simulink library "hil14_mdl_lib"  (Simulink 7.0)
values from neighbouring files (symbols this model uses):
  air =     [ws.mat]
  amb =     [ws.mat]
  cylinder =     [ws.mat]
  fuel =     [ws.mat]
  im =     [ws.mat]
  MDL =     [ws.mat]
  mph_per_m_per_sec = 2.23713646532    [ws.mat]
  tc =     [ws.mat]
  trans =     [ws.mat]
  veh =     [ws.mat]
  whl =     [ws.mat]
libraries: ni_annotations_lib x13
settings Model: Creator=Eric Bradley  LastModifiedBy=Eric Bradley

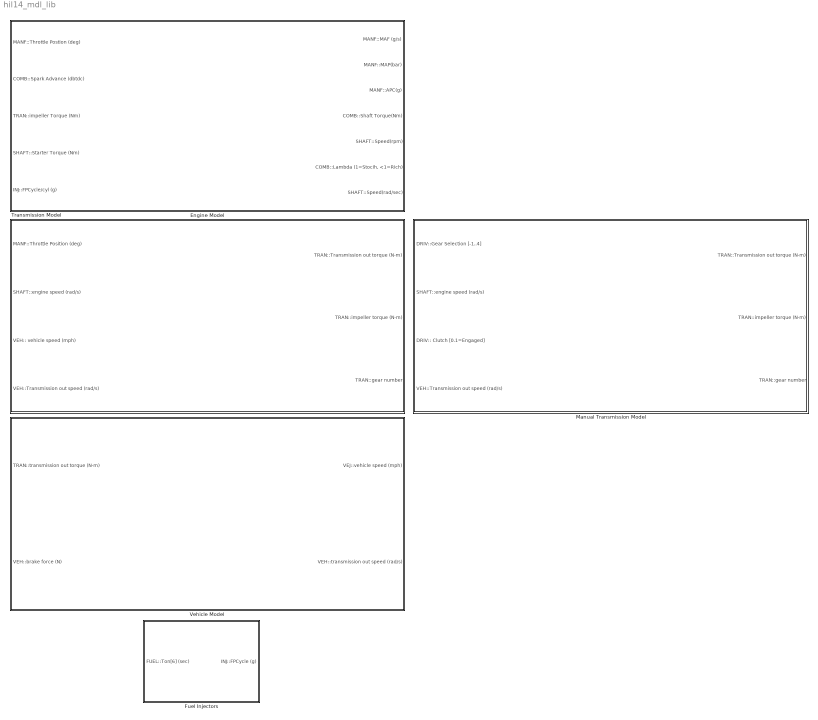
== system hil14_mdl_lib ==
  Engine Model : Subsystem  mask{iname='engine.jpg'}
      mask prompts: iname "Image"
      mask init:
      | blk = gcb;
      | 
      | p = get_param(blk,'Position');
      | 
      | wd = p(3)-p(1);
      | ht = p(4)-p(2);
      | 
      | ar = wd/ht;
      | 
      | img = imread(iname);
      | ii = imfinfo(iname);
      | 
      | iar = ii.Width/ii.Height;
      | 
      | scale = 0.125;
      settings: OpenFcn=open_system(gcb,'Force')
      mask Display: image(img, [0.5-ii.Width/wd*scale/2, 0.5-ii.Height/ht*scale/2, ii.Width/wd*scale,ii.Height/ht*scale]);
  Fuel Injectors : Subsystem  mask{iname='pfi.jpg', scale=0.125}
      mask prompts: iname "Image"
      mask init:
      | blk = gcb;
      | 
      | p = get_param(blk,'Position');
      | 
      | wd = p(3)-p(1);
      | ht = p(4)-p(2);
      | 
      | ar = wd/ht;
      | 
      | img = imread(iname);
      | ii = imfinfo(iname);
      | 
      | iar = ii.Width/ii.Height;
      settings: OpenFcn=open_system(gcb,'Force')
      mask Display: image(img, [0.5-ii.Width/wd*scale/2, 0.5-ii.Height/ht*scale/2, ii.Width/wd*scale,ii.Height/ht*scale]);
  Manual Transmission Model : Subsystem  mask{iname='Manual_Transmission.png', scale=0.55}
      mask prompts: iname "Image"
      mask init:
      | blk = gcb;
      | 
      | p = get_param(blk,'Position');
      | 
      | wd = p(3)-p(1);
      | ht = p(4)-p(2);
      | 
      | ar = wd/ht;
      | 
      | img = imread(iname);
      | ii = imfinfo(iname);
      | 
      | iar = ii.Width/ii.Height;
      settings: OpenFcn=open_system(gcb,'Force')
      mask Display: image(img, [0.5-ii.Width/wd*scale/2, 0.5-ii.Height/ht*scale/2, ii.Width/wd*scale,ii.Height/ht*scale]);
  Transmission Model : Subsystem  mask{iname='tran.jpg', scale=0.375}
      mask prompts: iname "Image"
      mask init:
      | blk = gcb;
      | 
      | p = get_param(blk,'Position');
      | 
      | wd = p(3)-p(1);
      | ht = p(4)-p(2);
      | 
      | ar = wd/ht;
      | 
      | img = imread(iname);
      | ii = imfinfo(iname);
      | 
      | iar = ii.Width/ii.Height;
      settings: OpenFcn=open_system(gcb,'Force')
      mask Display: image(img, [0.5-ii.Width/wd*scale/2, 0.5-ii.Height/ht*scale/2, ii.Width/wd*scale,ii.Height/ht*scale]);
  Vehicle Model : Subsystem  mask{iname='veh.jpg', scale=0.5}
      mask prompts: iname "Image"
      mask init:
      | blk = gcb;
      | 
      | p = get_param(blk,'Position');
      | 
      | wd = p(3)-p(1);
      | ht = p(4)-p(2);
      | 
      | ar = wd/ht;
      | 
      | img = imread(iname);
      | ii = imfinfo(iname);
      | 
      | iar = ii.Width/ii.Height;
      settings: OpenFcn=open_system(gcb,'Force')
      mask Display: image(img, [0.5-ii.Width/wd*scale/2, 0.5-ii.Height/ht*scale/2, ii.Width/wd*scale,ii.Height/ht*scale]);

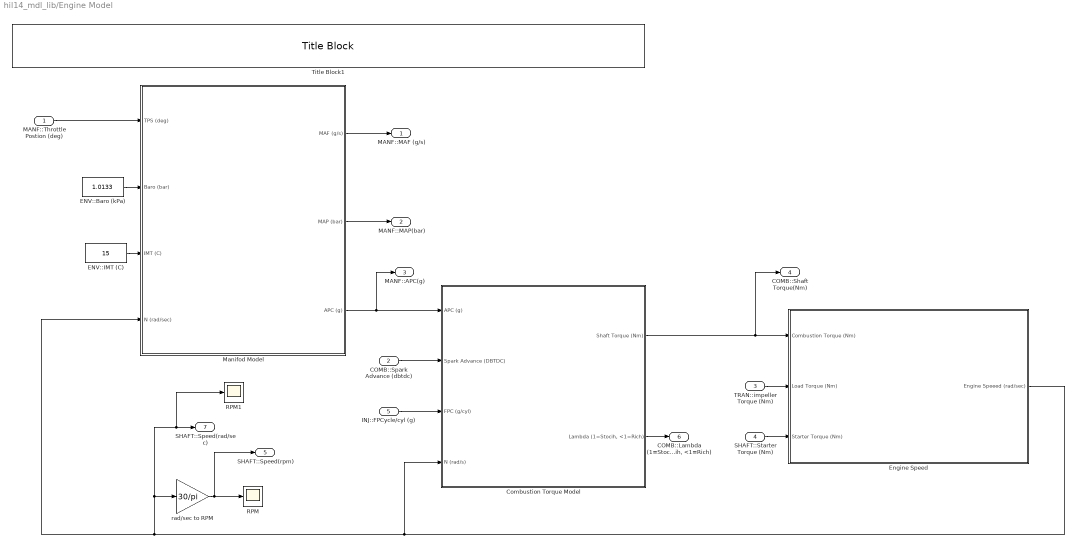
== system hil14_mdl_lib/Engine Model ==
  MANF::Throttle Postion (deg) : Inport  OutDataType=sfix(16)  OutScaling=2^0
  COMB::Spark Advance (dbtdc) : Inport  Port=2  PortDimensions=6  OutDataType=sfix(16)  OutScaling=2^0
  TRAN::impeller Torque (Nm) : Inport  Port=3  OutDataType=sfix(16)  OutScaling=2^0
  SHAFT::Starter Torque (Nm) : Inport  Port=4  OutDataType=sfix(16)  OutScaling=2^0
  INJ::FPCycle/cyl (g) : Inport  Port=5  OutDataType=sfix(16)  OutScaling=2^0
  Combustion Torque Model : Subsystem  mask{iname='cylinder.jpg'}
      mask prompts: iname "Image"
      mask init:
      | blk = gcb;
      | 
      | p = get_param(blk,'Position');
      | 
      | wd = p(3)-p(1);
      | ht = p(4)-p(2);
      | 
      | ar = wd/ht;
      | 
      | img = imread(iname);
      | ii = imfinfo(iname);
      | 
      | iar = ii.Width/ii.Height;
      settings: OpenFcn=open_system(gcb,'Force')
      mask Display: image(img, [0.5-ii.Width/wd*0.125/2, 0.5-ii.Height/ht*0.125/2, ii.Width/wd*0.125,ii.Height/ht*0.125]);
  ENV::Baro (kPa) : Constant  Value=1.0133  OutDataType=sfix(16)  OutScaling=2^0
  ENV::IMT (C) : Constant  Value=15  OutDataType=sfix(16)  OutScaling=2^0
  Engine Speed : Subsystem  mask{iname='piston.jpg'}
      mask prompts: iname "Image"
      mask init:
      | blk = gcb;
      | 
      | p = get_param(blk,'Position');
      | 
      | wd = p(3)-p(1);
      | ht = p(4)-p(2);
      | 
      | ar = wd/ht;
      | 
      | img = imread(iname);
      | ii = imfinfo(iname);
      | 
      | iar = ii.Width/ii.Height;
      settings: OpenFcn=open_system(gcb,'Force')
      mask Display: image(img, [0.5-ii.Width/wd*0.5/2, 0.5-ii.Height/ht*0.5/2, ii.Width/wd*0.5,ii.Height/ht*0.5]);
  Manifod Model : Subsystem  mask{iname='intake_manifold.jpg'}
      mask prompts: iname "Image"
      mask init:
      | blk = gcb;
      | 
      | p = get_param(blk,'Position');
      | 
      | wd = p(3)-p(1);
      | ht = p(4)-p(2);
      | 
      | ar = wd/ht;
      | 
      | img = imread(iname);
      | ii = imfinfo(iname);
      | 
      | iar = ii.Width/ii.Height;
      settings: OpenFcn=open_system(gcb,'Force')
      mask Display: image(img, [0.5-ii.Width/wd*0.25/2, 0.5-ii.Height/ht*0.25/2, ii.Width/wd*0.25,ii.Height/ht*0.25]);
  RPM : Scope
      settings: YMin=1100  YMax=2200  SaveName=ScopeData8
  RPM1 : Scope
      settings: YMin=1100  YMax=2200  SaveName=ScopeData14
  Title Block1 : ni_annotations_lib/Title Block  SystemSampleTime=-1  tx_title=get_param(gcs,'Name')
  rad/sec to RPM : Gain  Gain=30/pi  ParameterDataType=sfix(16)  ParameterScaling=2^0  OutDataType=sfix(16)  OutScaling=2^0
  MANF::MAF (g/s) : Outport  OutDataType=sfix(16)  OutScaling=2^0
  MANF::MAP(bar) : Outport  Port=2  OutDataType=sfix(16)  OutScaling=2^0
  MANF::APC(g) : Outport  Port=3  OutDataType=sfix(16)  OutScaling=2^0
  COMB::Shaft Torque(Nm) : Outport  Port=4  OutDataType=sfix(16)  OutScaling=2^0
  SHAFT::Speed(rpm) : Outport  Port=5  OutDataType=sfix(16)  OutScaling=2^0
  "COMB::Lambda (1=Stocih, <1=Rich)" : Outport  Port=6  OutDataType=sfix(16)  OutScaling=2^0
  SHAFT::Speed(rad/sec) : Outport  Port=7  OutDataType=sfix(16)  OutScaling=2^0
  wires:
  INJ::FPCycle/cyl (g)/1 -> Combustion Torque Model/3(FPC (g/cyl))
  SHAFT::Starter Torque (Nm)/1 -> Engine Speed/3(Starter Torque (Nm))
  TRAN::impeller Torque (Nm)/1 -> Engine Speed/2(Load Torque (Nm))
  COMB::Spark Advance (dbtdc)/1 -> Combustion Torque Model/2(Spark Advance (DBTDC))
  Combustion Torque Model/2("Lambda (1=Stocih, <1=Rich)") -> "COMB::Lambda (1=Stocih, <1=Rich)"/1
  MANF::Throttle Postion (deg)/1 -> Manifod Model/1(TPS (deg))
  Engine Speed/1(Engine Speeed (rad/sec)) -> Combustion Torque Model/4(N (rad/s)), RPM1/1, SHAFT::Speed(rad/sec)/1, rad/sec to RPM/1, Manifod Model/4(N (rad/sec))
  rad/sec to RPM/1 -> SHAFT::Speed(rpm)/1, RPM/1
  Combustion Torque Model/1(Shaft Torque (Nm)) -> COMB::Shaft Torque(Nm)/1, Engine Speed/1(Combustion Torque (Nm))
  Manifod Model/3(APC (g)) -> Combustion Torque Model/1(APC (g)), MANF::APC(g)/1
  Manifod Model/2(MAP (bar)) -> MANF::MAP(bar)/1
  Manifod Model/1(MAF (g/s)) -> MANF::MAF (g/s)/1
  ENV::IMT (C)/1 -> Manifod Model/3(IMT (C))
  ENV::Baro (kPa)/1 -> Manifod Model/2(Baro (bar))

== system hil14_mdl_lib/Fuel Injectors ==
  FUEL::Ton[6] (sec) : Inport  PortDimensions=6  OutDataType=sfix(16)  OutScaling=2^0
  Injector Curve : Lookup  InputValues=MDL.ECU_ENGINE.InjectionTime.v(14,:)'  Table=MDL.ECU_ENGINE.InjectionTime.y*1000  LookUpMeth=Interpolation-Use End Values  OutDataTypeMode=double  OutDataType=sfix(16)  OutScaling=2^0
  Sum of Elements : Sum  Inputs=+  OutDataType=sfix(16)  OutScaling=2^-10
  Title Block1 : ni_annotations_lib/Title Block  SystemSampleTime=-1  tx_title=get_param(gcs,'Name')
  INJ::FPCycle (g) : Outport  OutDataType=sfix(16)  OutScaling=2^0
  wires:
  Sum of Elements/1 -> INJ::FPCycle (g)/1
  Injector Curve/1 -> Sum of Elements/1
  FUEL::Ton[6] (sec)/1 -> Injector Curve/1

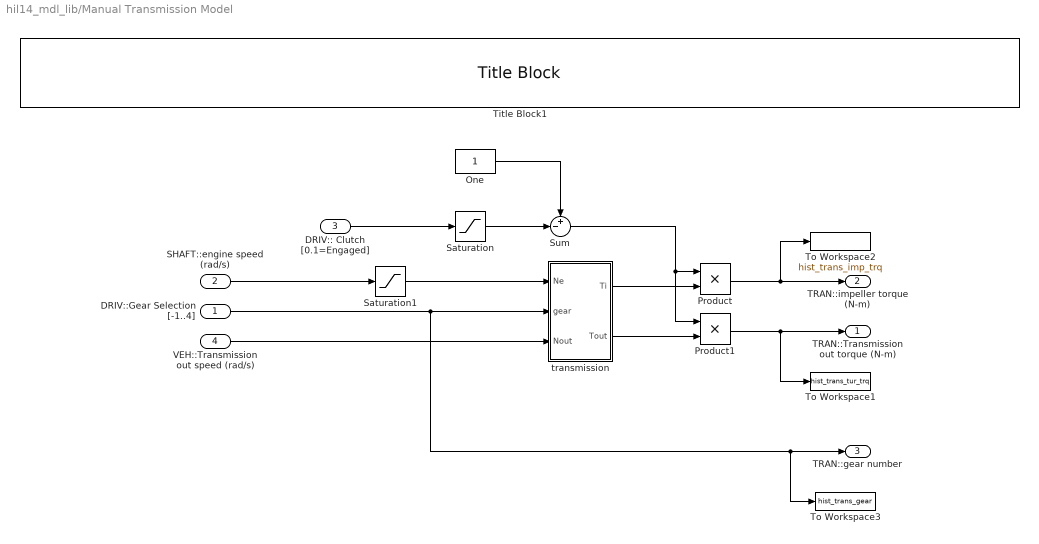
== system hil14_mdl_lib/Manual Transmission Model ==
  DRIV::Gear Selection [-1..4] : Inport  OutDataType=sfix(16)  OutScaling=2^0
  SHAFT::engine speed (rad/s) : Inport  Port=2  OutDataType=sfix(16)  OutScaling=2^0
  DRIV:: Clutch [0.1=Engaged] : Inport  Port=3  OutDataType=sfix(16)  OutScaling=2^0
  VEH::Transmission out speed (rad/s) : Inport  Port=4  OutDataType=sfix(16)  OutScaling=2^0
  One : Constant  OutDataType=sfix(16)  OutScaling=2^0
  Product : Product  OutDataType=sfix(16)  OutScaling=2^0  RndMeth=Zero
  Product1 : Product  OutDataType=sfix(16)  OutScaling=2^0  RndMeth=Zero
  Saturation : Saturate  UpperLimit=1  LowerLimit=0  OutDataType=sfix(16)  OutScaling=2^0
  Saturation1 : Saturate  UpperLimit=inf  LowerLimit=2*pi/60  OutDataType=sfix(16)  OutScaling=2^0
  Sum : Sum  Inputs=+-|  OutDataType=sfix(16)  OutScaling=2^0
  Title Block1 : ni_annotations_lib/Title Block  SystemSampleTime=-1  tx_title=get_param(gcs,'Name')
  To Workspace1 : ToWorkspace  VariableName=hist_trans_tur_trq  SampleTime=-1  SaveFormat=Array
      settings: MaxDataPoints=hist_sample_size
  To Workspace2 : ToWorkspace  VariableName=hist_trans_imp_trq  SampleTime=-1  SaveFormat=Array
      settings: MaxDataPoints=hist_sample_size
  To Workspace3 : ToWorkspace  VariableName=hist_trans_gear  SampleTime=-1  SaveFormat=Array
      settings: MaxDataPoints=hist_sample_size
  transmission : Subsystem
  TRAN::Transmission out torque (N-m) : Outport  InitialOutput=0
  TRAN::impeller torque (N-m) : Outport  Port=2  InitialOutput=0
  TRAN::gear number : Outport  Port=3  InitialOutput=0
  wires:
  Saturation1/1 -> transmission/1(Ne)
  Sum/1 -> Product1/1, Product/1
  One/1 -> Sum/1
  Saturation/1 -> Sum/2
  Product1/1 -> To Workspace1/1, TRAN::Transmission out torque (N-m)/1
  transmission/2(Tout) -> Product1/2
  transmission/1(Ti) -> Product/2
  Product/1 -> To Workspace2/1, TRAN::impeller torque (N-m)/1
  DRIV:: Clutch [0.1=Engaged]/1 -> Saturation/1
  DRIV::Gear Selection [-1..4]/1 -> To Workspace3/1, TRAN::gear number/1, transmission/2(gear)
  VEH::Transmission out speed (rad/s)/1 -> transmission/3(Nout)
  SHAFT::engine speed (rad/s)/1 -> Saturation1/1

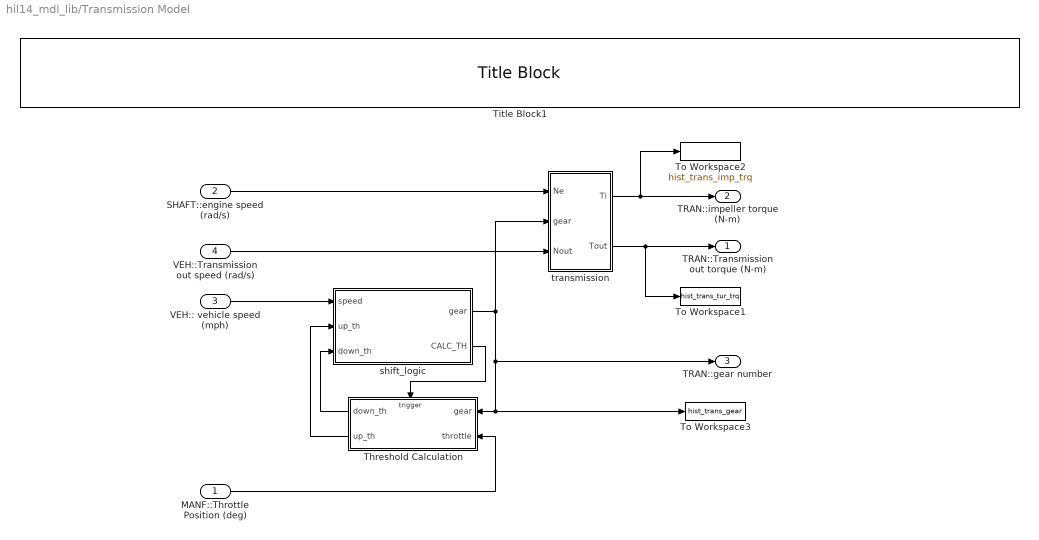
== system hil14_mdl_lib/Transmission Model ==
  MANF::Throttle Position (deg) : Inport  OutDataType=sfix(16)  OutScaling=2^0
  SHAFT::engine speed (rad/s) : Inport  Port=2  OutDataType=sfix(16)  OutScaling=2^0
  VEH:: vehicle speed (mph) : Inport  Port=3  OutDataType=sfix(16)  OutScaling=2^0
  VEH::Transmission out speed (rad/s) : Inport  Port=4  OutDataType=sfix(16)  OutScaling=2^0
  Threshold Calculation : Subsystem  Orientation=left  TreatAsAtomicUnit=on
  Title Block1 : ni_annotations_lib/Title Block  SystemSampleTime=-1  tx_title=get_param(gcs,'Name')
  To Workspace1 : ToWorkspace  VariableName=hist_trans_tur_trq  SampleTime=-1  SaveFormat=Array
      settings: MaxDataPoints=hist_sample_size
  To Workspace2 : ToWorkspace  VariableName=hist_trans_imp_trq  SampleTime=-1  SaveFormat=Array
      settings: MaxDataPoints=hist_sample_size
  To Workspace3 : ToWorkspace  VariableName=hist_trans_gear  SampleTime=-1  SaveFormat=Array
      settings: MaxDataPoints=hist_sample_size
  shift_logic : Stateflow chart
  transmission : Subsystem
  TRAN::Transmission out torque (N-m) : Outport  InitialOutput=0
  TRAN::impeller torque (N-m) : Outport  Port=2  InitialOutput=0
  TRAN::gear number : Outport  Port=3  InitialOutput=0
  wires:
  VEH::Transmission out speed (rad/s)/1 -> transmission/3(Nout)
  VEH:: vehicle speed (mph)/1 -> shift_logic/1(speed)
  transmission/1(Ti) -> TRAN::impeller torque (N-m)/1, To Workspace2/1
  MANF::Throttle Position (deg)/1 -> Threshold Calculation/2(throttle)
  SHAFT::engine speed (rad/s)/1 -> transmission/1(Ne)
  transmission/2(Tout) -> TRAN::Transmission out torque (N-m)/1, To Workspace1/1
  Threshold Calculation/1(down_th) -> shift_logic/3(down_th)
  Threshold Calculation/2(up_th) -> shift_logic/2(up_th)
  shift_logic/1(gear) -> transmission/2(gear), Threshold Calculation/1(gear), To Workspace3/1, TRAN::gear number/1
  shift_logic/2(CALC_TH) -> Threshold Calculation/Trigger

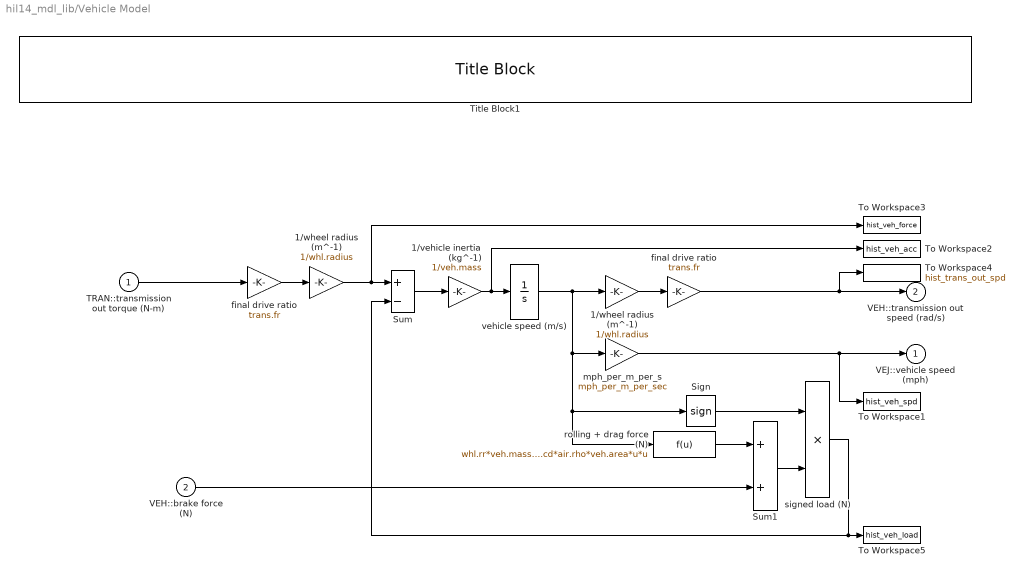
== system hil14_mdl_lib/Vehicle Model ==
  TRAN::transmission out torque (N-m) : Inport  OutDataType=sfix(16)  OutScaling=2^0
  VEH::brake force (N) : Inport  Port=2  OutDataType=sfix(16)  OutScaling=2^0
  1/vehicle inertia (kg^-1) : Gain  Gain=1/veh.mass  ParameterDataType=sfix(16)  ParameterScaling=2^0  OutDataType=sfix(16)  OutScaling=2^0  SaturateOnIntegerOverflow=on
  1/wheel radius (m^-1) : Gain  Gain=1/whl.radius  ParameterDataType=sfix(16)  ParameterScaling=2^0  OutDataType=sfix(16)  OutScaling=2^0  SaturateOnIntegerOverflow=on
  "1/wheel radius (m^-1) " : Gain  Gain=1/whl.radius  ParameterDataType=sfix(16)  ParameterScaling=2^0  OutDataType=sfix(16)  OutScaling=2^0  SaturateOnIntegerOverflow=on
  Sign : Signum
  Sum : Sum  Inputs=+-  OutDataType=sfix(16)  OutScaling=2^0  SaturateOnIntegerOverflow=on  InputSameDT=on
  Sum1 : Sum  OutDataType=sfix(16)  OutScaling=2^0  SaturateOnIntegerOverflow=on  InputSameDT=on
  Title Block1 : ni_annotations_lib/Title Block  SystemSampleTime=-1  tx_title=get_param(gcs,'Name')
  To Workspace1 : ToWorkspace  VariableName=hist_veh_spd  SampleTime=-1  SaveFormat=Array
      settings: MaxDataPoints=hist_sample_size
  To Workspace2 : ToWorkspace  VariableName=hist_veh_acc  SampleTime=-1  SaveFormat=Array
      settings: MaxDataPoints=hist_sample_size
  To Workspace3 : ToWorkspace  VariableName=hist_veh_force  SampleTime=-1  SaveFormat=Array
      settings: MaxDataPoints=hist_sample_size
  To Workspace4 : ToWorkspace  VariableName=hist_trans_out_spd  SampleTime=-1  SaveFormat=Array
      settings: MaxDataPoints=hist_sample_size
  To Workspace5 : ToWorkspace  VariableName=hist_veh_load  SampleTime=-1  SaveFormat=Array
      settings: MaxDataPoints=hist_sample_size
  final drive ratio : Gain  Gain=trans.fr  ParameterDataType=sfix(16)  ParameterScaling=2^0  OutDataType=sfix(16)  OutScaling=2^0  SaturateOnIntegerOverflow=on
  "final drive ratio " : Gain  Gain=trans.fr  ParameterDataType=sfix(16)  ParameterScaling=2^0  OutDataType=sfix(16)  OutScaling=2^0  SaturateOnIntegerOverflow=on
  mph_per_m_per_s : Gain  Gain=mph_per_m_per_sec  ParameterDataType=sfix(16)  ParameterScaling=2^0  OutDataType=sfix(16)  OutScaling=2^0  SaturateOnIntegerOverflow=on
  rolling + drag force (N) : Fcn  Expr=whl.rr*veh.mass*9.81 + 1/2*veh.cd*air.rho*veh.area*u*u
  signed load (N) : Product  OutDataType=sfix(16)  OutScaling=2^0  SaturateOnIntegerOverflow=on  InputSameDT=on
  vehicle speed (m/s) : Integrator  LowerSaturationLimit=0  ZeroCross=off
  VEJ::vehicle speed (mph) : Outport  InitialOutput=0
  VEH::transmission out speed (rad/s) : Outport  Port=2  InitialOutput=0
  wires:
  mph_per_m_per_s/1 -> To Workspace1/1, VEJ::vehicle speed (mph)/1
  "1/wheel radius (m^-1) "/1 -> "final drive ratio "/1
  signed load (N)/1 -> Sum/2, To Workspace5/1
  vehicle speed (m/s)/1 -> mph_per_m_per_s/1, Sign/1, rolling + drag force (N)/1, "1/wheel radius (m^-1) "/1
  1/vehicle inertia (kg^-1)/1 -> To Workspace2/1, vehicle speed (m/s)/1
  Sum/1 -> 1/vehicle inertia (kg^-1)/1
  1/wheel radius (m^-1)/1 -> To Workspace3/1, Sum/1
  final drive ratio/1 -> 1/wheel radius (m^-1)/1
  TRAN::transmission out torque (N-m)/1 -> final drive ratio/1
  Sign/1 -> signed load (N)/1
  rolling + drag force (N)/1 -> Sum1/1
  Sum1/1 -> signed load (N)/2
  VEH::brake force (N)/1 -> Sum1/2
  "final drive ratio "/1 -> To Workspace4/1, VEH::transmission out speed (rad/s)/1

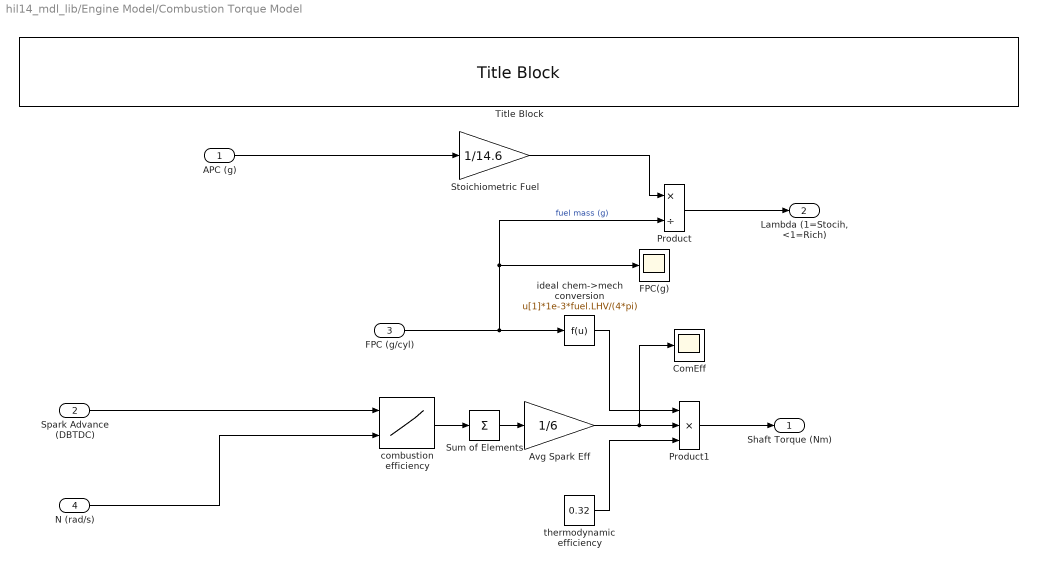
== system hil14_mdl_lib/Engine Model/Combustion Torque Model ==
  APC (g) : Inport  OutDataType=sfix(16)  OutScaling=2^0
  Spark Advance (DBTDC) : Inport  Port=2  OutDataType=sfix(16)  OutScaling=2^0
  FPC (g/cyl) : Inport  Port=3  OutDataType=sfix(16)  OutScaling=2^0
  N (rad/s) : Inport  Port=4  PortDimensions=1  OutDataType=sfix(16)  OutScaling=2^0
  Avg Spark Eff : Gain  Gain=1/6  ParameterDataType=sfix(16)  ParameterScaling=2^0  OutDataType=sfix(16)  OutScaling=2^0  SaturateOnIntegerOverflow=on
  ComEff : Scope
      settings: SaveName=ScopeData10
  FPC(g) : Scope
      settings: SaveName=ScopeData7
  Product : Product  Inputs=*/  OutDataType=sfix(16)  OutScaling=2^0  SaturateOnIntegerOverflow=on
  Product1 : Product  Inputs=3  OutDataType=sfix(16)  OutScaling=2^0  SaturateOnIntegerOverflow=on
  Stoichiometric Fuel : Gain  Gain=1/14.6  ParameterDataType=sfix(16)  ParameterScaling=2^0  OutDataType=sfix(16)  OutScaling=2^0  SaturateOnIntegerOverflow=on
  Sum of Elements : Sum  Inputs=+  OutDataType=sfix(16)  OutScaling=2^-10
  Title Block : ni_annotations_lib/Title Block  SystemSampleTime=-1  tx_title=get_param(gcs,'Name')
  combustion efficiency : Lookup2D  RowIndex=cylinder.ce.spark_timing  ColumnIndex=cylinder.ce.rpm*pi/30  Table=cylinder.ce.table  LookUpMeth=Interpolation-Use End Values  OutDataType=sfix(16)  OutScaling=2^0  SaturateOnIntegerOverflow=on
  ideal chem->mech conversion : Fcn  Expr=u[1]*1e-3*fuel.LHV/(4*pi)
  thermodynamic efficiency : Constant  Value=0.32  OutDataType=sfix(16)  OutScaling=2^0
  Shaft Torque (Nm) : Outport  OutDataType=sfix(16)  OutScaling=2^0
  "Lambda (1=Stocih, <1=Rich)" : Outport  Port=2  OutDataType=sfix(16)  OutScaling=2^0
  wires:
  Avg Spark Eff/1 -> ComEff/1, Product1/2
  Sum of Elements/1 -> Avg Spark Eff/1
  Product/1 -> "Lambda (1=Stocih, <1=Rich)"/1
  Stoichiometric Fuel/1 -> Product/1
  APC (g)/1 -> Stoichiometric Fuel/1
  Product1/1 -> Shaft Torque (Nm)/1
  thermodynamic efficiency/1 -> Product1/3
  ideal chem->mech conversion/1 -> Product1/1
  combustion efficiency/1 -> Sum of Elements/1
  FPC (g/cyl)/1 -> Product/2, FPC(g)/1, ideal chem->mech conversion/1  "fuel mass (g)"
  Spark Advance (DBTDC)/1 -> combustion efficiency/1
  N (rad/s)/1 -> combustion efficiency/2

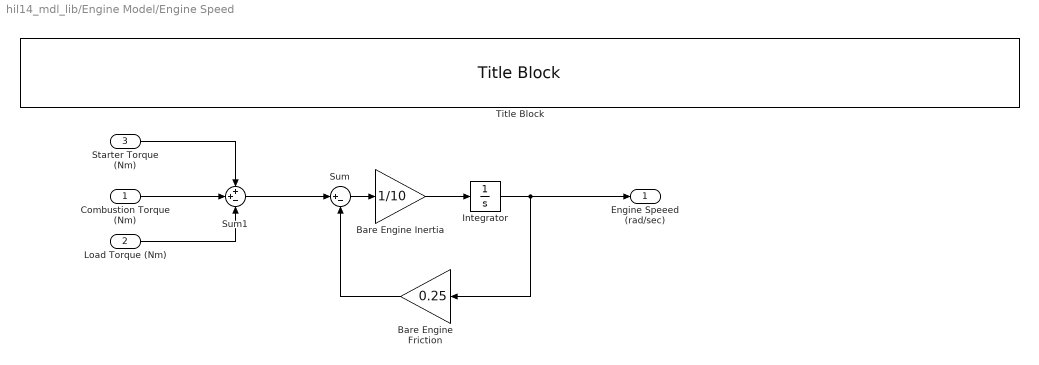
== system hil14_mdl_lib/Engine Model/Engine Speed ==
  Combustion Torque (Nm) : Inport  OutDataType=sfix(16)  OutScaling=2^0
  Load Torque (Nm) : Inport  Port=2  OutDataType=sfix(16)  OutScaling=2^0
  Starter Torque (Nm) : Inport  Port=3  OutDataType=sfix(16)  OutScaling=2^0
  Bare Engine Friction : Gain  Orientation=left  Gain=0.25  ParameterDataType=sfix(16)  ParameterScaling=2^0  OutDataType=sfix(16)  OutScaling=2^0
  Bare Engine Inertia : Gain  Gain=1/10  ParameterDataType=sfix(16)  ParameterScaling=2^0  OutDataType=sfix(16)  OutScaling=2^0
  Integrator : Integrator  InitialCondition=600*pi/30  LimitOutput=on  UpperSaturationLimit=1000  LowerSaturationLimit=0
  Sum : Sum  Inputs=|+-  OutDataType=sfix(16)  OutScaling=2^0
  Sum1 : Sum  Inputs=++-  OutDataType=sfix(16)  OutScaling=2^0
  Title Block : ni_annotations_lib/Title Block  SystemSampleTime=-1  tx_title=get_param(gcs,'Name')
  Engine Speeed (rad/sec) : Outport  OutDataType=sfix(16)  OutScaling=2^0
  wires:
  Starter Torque (Nm)/1 -> Sum1/1
  Sum1/1 -> Sum/1
  Combustion Torque (Nm)/1 -> Sum1/2
  Load Torque (Nm)/1 -> Sum1/3
  Bare Engine Friction/1 -> Sum/2
  Integrator/1 -> Bare Engine Friction/1, Engine Speeed (rad/sec)/1
  Bare Engine Inertia/1 -> Integrator/1
  Sum/1 -> Bare Engine Inertia/1

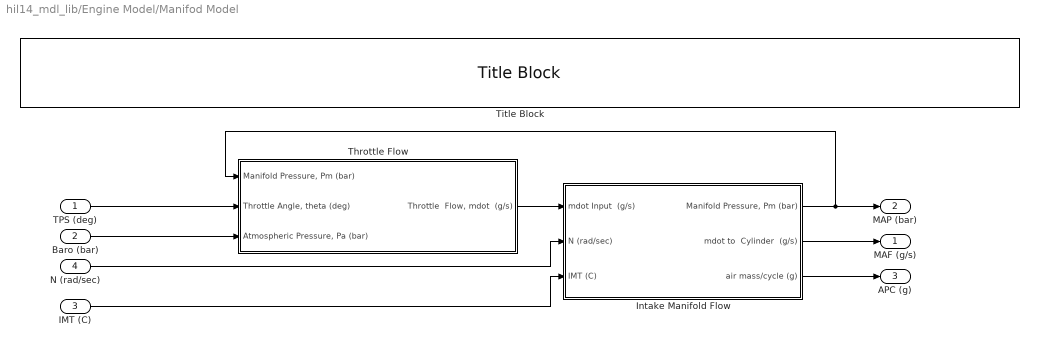
== system hil14_mdl_lib/Engine Model/Manifod Model ==
  TPS (deg) : Inport  OutDataType=sfix(16)  OutScaling=2^0
  Baro (bar) : Inport  Port=2  OutDataType=sfix(16)  OutScaling=2^0
  IMT (C) : Inport  Port=3  OutDataType=sfix(16)  OutScaling=2^0
  N (rad/sec) : Inport  Port=4  OutDataType=sfix(16)  OutScaling=2^0
  Intake Manifold Flow : Subsystem
  Throttle Flow : Subsystem
  Title Block : ni_annotations_lib/Title Block  SystemSampleTime=-1  tx_title=get_param(gcs,'Name')
  MAF (g/s) : Outport  OutDataType=sfix(16)  OutScaling=2^0
  MAP (bar) : Outport  Port=2  OutDataType=sfix(16)  OutScaling=2^0
  APC (g) : Outport  Port=3  OutDataType=sfix(16)  OutScaling=2^0
  wires:
  Intake Manifold Flow/1("Manifold Pressure, Pm (bar)") -> Throttle Flow/1("Manifold Pressure, Pm (bar)"), MAP (bar)/1
  Intake Manifold Flow/3(air mass/cycle (g)) -> APC (g)/1
  Intake Manifold Flow/2(mdot to  Cylinder  (g/s)) -> MAF (g/s)/1
  Throttle Flow/1("Throttle  Flow, mdot  (g/s)") -> Intake Manifold Flow/1(mdot Input  (g/s))
  Baro (bar)/1 -> Throttle Flow/3("Atmospheric Pressure, Pa (bar) ")
  N (rad/sec)/1 -> Intake Manifold Flow/2(N (rad/sec))
  IMT (C)/1 -> Intake Manifold Flow/3(IMT (C))
  TPS (deg)/1 -> Throttle Flow/2("Throttle Angle, theta (deg)")

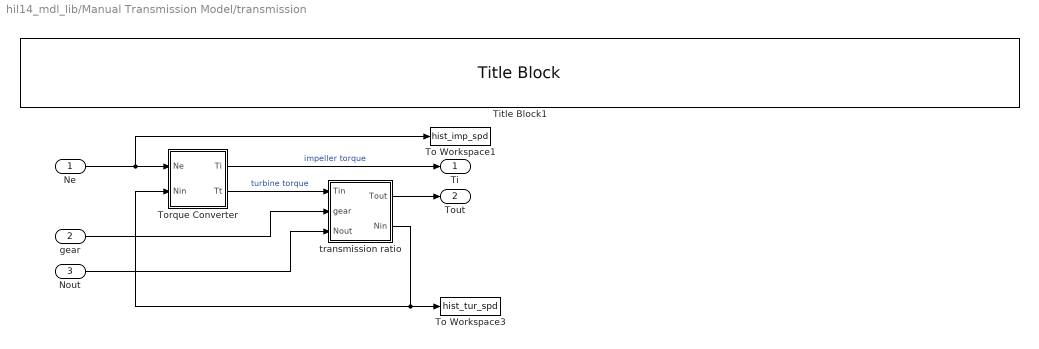
== system hil14_mdl_lib/Manual Transmission Model/transmission ==
  Ne : Inport  OutDataType=sfix(16)  OutScaling=2^0
  gear : Inport  Port=2  OutDataType=sfix(16)  OutScaling=2^0
  Nout : Inport  Port=3  OutDataType=sfix(16)  OutScaling=2^0
  Title Block1 : ni_annotations_lib/Title Block  SystemSampleTime=-1  tx_title=get_param(gcs,'Name')
  To Workspace1 : ToWorkspace  VariableName=hist_imp_spd  SampleTime=-1  SaveFormat=Array
      settings: MaxDataPoints=hist_sample_size
  To Workspace3 : ToWorkspace  VariableName=hist_tur_spd  SampleTime=-1  SaveFormat=Array
      settings: MaxDataPoints=hist_sample_size
  Torque Converter : Subsystem  mask(torque converter){speedratio=tc.tur_imp_ratio, Kfactor=tc.k_curve, Torkratio=tc.r_curve}
      mask prompts: speedratio "speed ratio"; Kfactor "K factor"; Torkratio "torque ratio"
      mask help: torque converter
      mask Help: Torque converter input and output torques are computed as a function of the input and output speeds
      mask Display: plot([cos([90:10:450]*pi/180),.63*cos([90:10:450]*pi/180),.63*cos([90:10:240]*pi/180),cos([240:10:300]*pi/180),.63*cos([300]*pi/180)],[sin([90:10:450]*pi/180),.63*sin([90:10:450]*pi/180)+.1,.63*sin([90:10:240]*pi/180)+.1,sin([240:10:300]*pi/180),.63*sin([300]*pi/180)+.1])
  transmission ratio : Subsystem
  Ti : Outport  InitialOutput=0
  Tout : Outport  Port=2  InitialOutput=0
  wires:
  Torque Converter/2(Tt) -> transmission ratio/1(Tin)  "turbine torque"
  transmission ratio/2(Nin) -> Torque Converter/2(Nin), To Workspace3/1
  Ne/1 -> Torque Converter/1(Ne), To Workspace1/1
  gear/1 -> transmission ratio/2(gear)
  Nout/1 -> transmission ratio/3(Nout)
  Torque Converter/1(Ti) -> Ti/1  "impeller torque"
  transmission ratio/1(Tout) -> Tout/1

== system hil14_mdl_lib/Transmission Model/Threshold Calculation ==
  gear : Inport  OutDataType=sfix(16)  OutScaling=2^0
  throttle : Inport  Port=2  OutDataType=sfix(16)  OutScaling=2^0
  run : TriggerPort  TriggerType=function-call  ZeroCross=off
  interp_down : Lookup2D  RowIndex=trans.downth  ColumnIndex=[1:4]  Table=trans.downtab  OutDataType=sfix(16)  OutScaling=2^-10  InputSameDT=on
  interp_up : Lookup2D  RowIndex=trans.upth  ColumnIndex=[1:4]  Table=trans.uptab  OutDataType=sfix(16)  OutScaling=2^-10  InputSameDT=on
  down_th : Outport
  up_th : Outport  Port=2
  wires:
  gear/1 -> interp_down/2, interp_up/2
  throttle/1 -> interp_down/1, interp_up/1
  interp_down/1 -> down_th/1
  interp_up/1 -> up_th/1

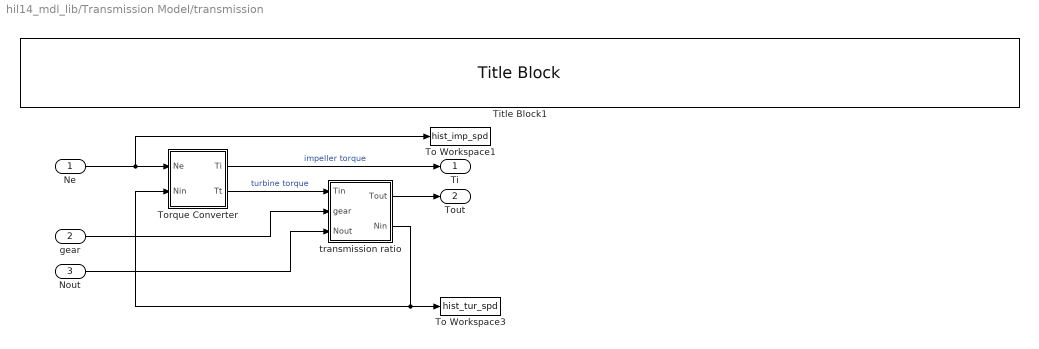
== system hil14_mdl_lib/Transmission Model/transmission ==
  Ne : Inport  OutDataType=sfix(16)  OutScaling=2^0
  gear : Inport  Port=2  OutDataType=sfix(16)  OutScaling=2^0
  Nout : Inport  Port=3  OutDataType=sfix(16)  OutScaling=2^0
  Title Block1 : ni_annotations_lib/Title Block  SystemSampleTime=-1  tx_title=get_param(gcs,'Name')
  To Workspace1 : ToWorkspace  VariableName=hist_imp_spd  SampleTime=-1  SaveFormat=Array
      settings: MaxDataPoints=hist_sample_size
  To Workspace3 : ToWorkspace  VariableName=hist_tur_spd  SampleTime=-1  SaveFormat=Array
      settings: MaxDataPoints=hist_sample_size
  Torque Converter : Subsystem  mask(torque converter){speedratio=tc.tur_imp_ratio, Kfactor=tc.k_curve, Torkratio=tc.r_curve}
      mask prompts: speedratio "speed ratio"; Kfactor "K factor"; Torkratio "torque ratio"
      mask help: torque converter
      mask Help: Torque converter input and output torques are computed as a function of the input and output speeds
      mask Display: plot([cos([90:10:450]*pi/180),.63*cos([90:10:450]*pi/180),.63*cos([90:10:240]*pi/180),cos([240:10:300]*pi/180),.63*cos([300]*pi/180)],[sin([90:10:450]*pi/180),.63*sin([90:10:450]*pi/180)+.1,.63*sin([90:10:240]*pi/180)+.1,sin([240:10:300]*pi/180),.63*sin([300]*pi/180)+.1])
  transmission ratio : Subsystem
  Ti : Outport  InitialOutput=0
  Tout : Outport  Port=2  InitialOutput=0
  wires:
  Torque Converter/2(Tt) -> transmission ratio/1(Tin)  "turbine torque"
  transmission ratio/2(Nin) -> Torque Converter/2(Nin), To Workspace3/1
  Ne/1 -> Torque Converter/1(Ne), To Workspace1/1
  gear/1 -> transmission ratio/2(gear)
  Nout/1 -> transmission ratio/3(Nout)
  Torque Converter/1(Ti) -> Ti/1  "impeller torque"
  transmission ratio/1(Tout) -> Tout/1

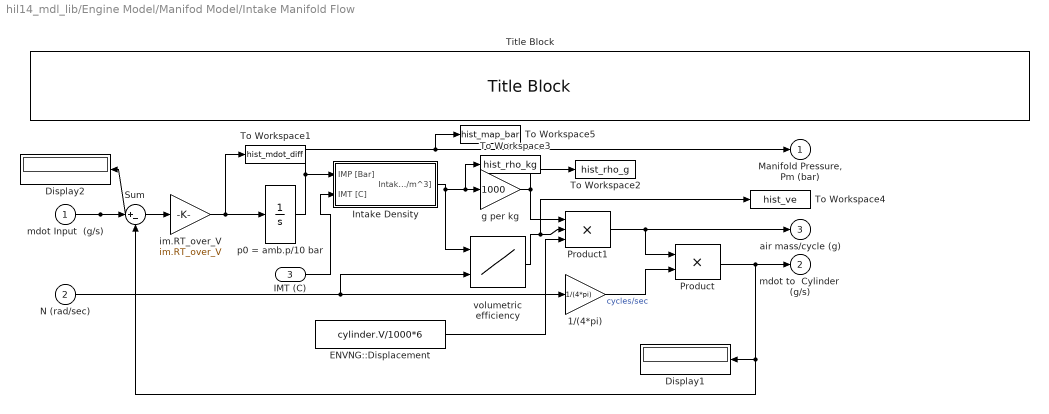
== system hil14_mdl_lib/Engine Model/Manifod Model/Intake Manifold Flow ==
  mdot Input  (g/s) : Inport  OutDataType=sfix(16)  OutScaling=2^0
  N (rad/sec) : Inport  Port=2  OutDataType=sfix(16)  OutScaling=2^0
  IMT (C) : Inport  Port=3  OutDataType=sfix(16)  OutScaling=2^0
  1/(4*pi) : Gain  Gain=1/(4*pi)  ParameterDataType=sfix(16)  ParameterScaling=2^0  OutDataType=sfix(16)  OutScaling=2^0  SaturateOnIntegerOverflow=on
  Display1 : Display
  Display2 : Display
  ENVNG::Displacement : Constant  Value=cylinder.V/1000*6  OutDataType=sfix(16)  OutScaling=2^0
  Intake Density : Subsystem
  Product : Product  OutDataType=sfix(16)  OutScaling=2^0  SaturateOnIntegerOverflow=on
  Product1 : Product  Inputs=3  OutDataType=sfix(16)  OutScaling=2^0  SaturateOnIntegerOverflow=on
  Sum : Sum  Inputs=|+-  OutDataType=sfix(16)  OutScaling=2^0  SaturateOnIntegerOverflow=on  InputSameDT=on
  Title Block : ni_annotations_lib/Title Block  SystemSampleTime=-1  tx_title=get_param(gcs,'Name')
  To Workspace1 : ToWorkspace  VariableName=hist_mdot_diff  SampleTime=-1  SaveFormat=Array
      settings: MaxDataPoints=hist_sample_size
  To Workspace2 : ToWorkspace  VariableName=hist_rho_g  SampleTime=-1  SaveFormat=Array
      settings: MaxDataPoints=hist_sample_size
  To Workspace3 : ToWorkspace  VariableName=hist_rho_kg  SampleTime=-1  SaveFormat=Array
      settings: MaxDataPoints=hist_sample_size
  To Workspace4 : ToWorkspace  VariableName=hist_ve  SampleTime=-1  SaveFormat=Array
      settings: MaxDataPoints=hist_sample_size
  To Workspace5 : ToWorkspace  VariableName=hist_map_bar  SampleTime=-1  SaveFormat=Array
      settings: MaxDataPoints=hist_sample_size
  g per kg : Gain  Gain=1000  ParameterDataType=sfix(16)  ParameterScaling=2^0  OutDataType=sfix(16)  OutScaling=2^0  SaturateOnIntegerOverflow=on
  im.RT_over_V : Gain  Gain=im.RT_over_V  ParameterDataType=sfix(16)  ParameterScaling=2^0  OutDataType=sfix(16)  OutScaling=2^0  SaturateOnIntegerOverflow=on
  p0 = amb.p/10 bar : Integrator  InitialCondition=amb.p*0.99  LimitOutput=on  UpperSaturationLimit=0.99*amb.p  LowerSaturationLimit=0.001*amb.p
  volumetric efficiency : Lookup2D  RowIndex=MDL.ENGINE.VolumetricEff.x  ColumnIndex=MDL.ENGINE.VolumetricEff.y  Table=0.7*MDL.ENGINE.VolumetricEff.v  LookUpMeth=Interpolation-Use End Values  OutDataType=sfix(16)  OutScaling=2^0  SaturateOnIntegerOverflow=on
  "Manifold Pressure, Pm (bar)" : Outport  InitialOutput=0
  mdot to  Cylinder  (g/s) : Outport  Port=2  InitialOutput=0
  air mass/cycle (g) : Outport  Port=3  InitialOutput=0
  wires:
  ENVNG::Displacement/1 -> Product1/3
  g per kg/1 -> To Workspace2/1, Product1/1
  Product1/1 -> Product/1, air mass/cycle (g)/1
  IMT (C)/1 -> Intake Density/2(IMT [C])
  Intake Density/1(Intake Density [Kg/m^3]) -> To Workspace3/1, g per kg/1, volumetric efficiency/1
  Product/1 -> Display1/1, Sum/2, mdot to  Cylinder  (g/s)/1
  1/(4*pi)/1 -> Product/2  "cycles/sec"
  volumetric efficiency/1 -> Product1/2, To Workspace4/1
  mdot Input  (g/s)/1 -> Display2/1, Sum/1
  im.RT_over_V/1 -> p0 = amb.p/10 bar/1, To Workspace1/1
  N (rad/sec)/1 -> 1/(4*pi)/1, volumetric efficiency/2
  Sum/1 -> im.RT_over_V/1
  p0 = amb.p/10 bar/1 -> To Workspace5/1, "Manifold Pressure, Pm (bar)"/1, Intake Density/1(IMP [Bar])

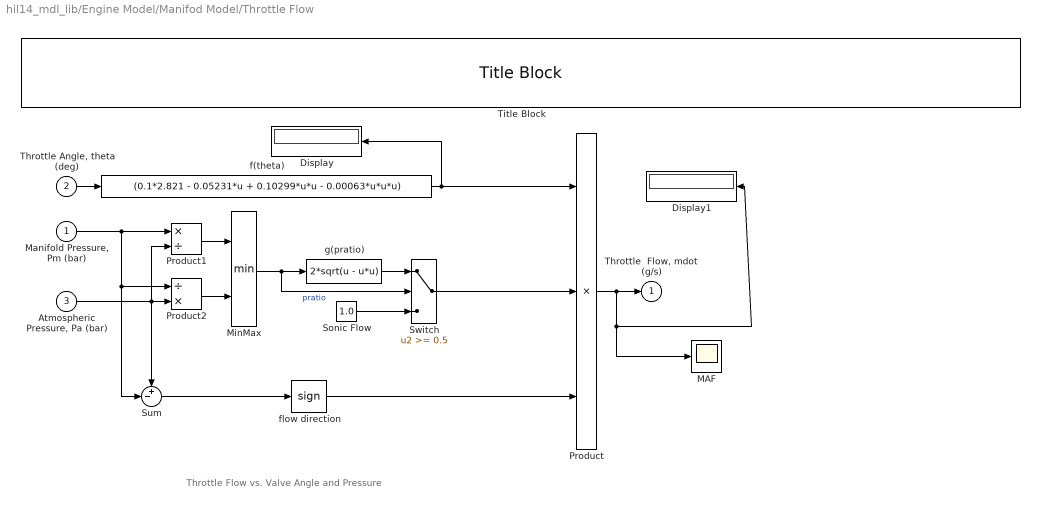
== system hil14_mdl_lib/Engine Model/Manifod Model/Throttle Flow ==
  note: Throttle Flow vs. Valve Angle and Pressure
  "Manifold Pressure, Pm (bar)" : Inport  OutDataType=sfix(16)  OutScaling=2^0
  "Throttle Angle, theta (deg)" : Inport  Port=2  OutDataType=sfix(16)  OutScaling=2^0
  "Atmospheric Pressure, Pa (bar) " : Inport  Port=3  OutDataType=sfix(16)  OutScaling=2^0
  Display : Display
  Display1 : Display
  MAF : Scope
      settings: YMin=1.5  YMax=8.5  SaveName=ScopeData11
  MinMax : MinMax  Inputs=2  SaturateOnIntegerOverflow=on  InputSameDT=on
  Product : Product  Inputs=3  OutDataType=sfix(16)  OutScaling=2^0  SaturateOnIntegerOverflow=on  InputSameDT=on
  Product1 : Product  Inputs=*/  OutDataType=sfix(16)  OutScaling=2^0  SaturateOnIntegerOverflow=on  InputSameDT=on
  Product2 : Product  Inputs=/*  OutDataType=sfix(16)  OutScaling=2^0  SaturateOnIntegerOverflow=on  InputSameDT=on
  "Sonic Flow " : Constant  Value=1.0  OutDataType=sfix(16)  OutScaling=2^0
  Sum : Sum  Inputs=+-|  OutDataType=sfix(16)  OutScaling=2^0  SaturateOnIntegerOverflow=on  InputSameDT=on
  Switch : Switch  Threshold=0.5  SaturateOnIntegerOverflow=on  InputSameDT=on
  Title Block : ni_annotations_lib/Title Block  SystemSampleTime=-1  tx_title=get_param(gcs,'Name')
  f(theta) : Fcn  Expr=(0.1*2.821 - 0.05231*u + 0.10299*u*u - 0.00063*u*u*u)
  flow direction : Signum
  g(pratio) : Fcn  Expr=2*sqrt(u - u*u)
  "Throttle  Flow, mdot  (g/s)" : Outport  InitialOutput=0
  wires:
  "Manifold Pressure, Pm (bar)"/1 -> Sum/2, Product2/1, Product1/1
  Product2/1 -> MinMax/2
  Product1/1 -> MinMax/1
  "Atmospheric Pressure, Pa (bar) "/1 -> Sum/1, Product2/2, Product1/2
  g(pratio)/1 -> Switch/1
  "Sonic Flow "/1 -> Switch/3
  Switch/1 -> Product/2
  flow direction/1 -> Product/3
  Sum/1 -> flow direction/1
  MinMax/1 -> Switch/2, g(pratio)/1  "pratio"
  "Throttle Angle, theta (deg)"/1 -> f(theta)/1
  Product/1 -> Display1/1, MAF/1, "Throttle  Flow, mdot  (g/s)"/1
  f(theta)/1 -> Display/1, Product/1

== system hil14_mdl_lib/Manual Transmission Model/transmission/Torque Converter ==
  Ne : Inport  OutDataType=sfix(16)  OutScaling=2^0
  Nin : Inport  Port=2  OutDataType=sfix(16)  OutScaling=2^0
  K factor : Lookup  InputValues=speedratio  Table=Kfactor  OutDataType=sfix(16)  OutScaling=2^0  SaturateOnIntegerOverflow=on
  Torque ratio : Lookup  InputValues=speedratio  Table=Torkratio  OutDataType=sfix(16)  OutScaling=2^0  SaturateOnIntegerOverflow=on
  impeller : Fcn  Expr=u^2
  quotient : Product  Inputs=*/  OutDataType=sfix(16)  OutScaling=2^0  SaturateOnIntegerOverflow=on  InputSameDT=on
  speed ratio : Product  Inputs=*/  OutDataType=sfix(16)  OutScaling=2^0  SaturateOnIntegerOverflow=on  InputSameDT=on
  turbine : Product  OutDataType=sfix(16)  OutScaling=2^0  SaturateOnIntegerOverflow=on  InputSameDT=on
  Ti : Outport  InitialOutput=0
  Tt : Outport  Port=2  InitialOutput=0
  wires:
  Nin/1 -> speed ratio/1
  Ne/1 -> quotient/1, speed ratio/2
  turbine/1 -> Tt/1
  impeller/1 -> Ti/1, turbine/1
  speed ratio/1 -> K factor/1, Torque ratio/1
  K factor/1 -> quotient/2
  quotient/1 -> impeller/1
  Torque ratio/1 -> turbine/2

== system hil14_mdl_lib/Manual Transmission Model/transmission/transmission ratio ==
  Tin : Inport  OutDataType=sfix(16)  OutScaling=2^0
  gear : Inport  Port=2  OutDataType=sfix(16)  OutScaling=2^0
  Nout : Inport  Orientation=left  Port=3  OutDataType=sfix(16)  OutScaling=2^0
  Abs : Abs  OutDataType=sfix(16)  OutScaling=2^0
  Abs1 : Abs  Orientation=left  OutDataType=sfix(16)  OutScaling=2^0
  Look-Up Table : Lookup  InputValues=[-1 0 1 2 3 4]  Table=[-2.393 0 2.393 1.450 1.000 0.677]  LookUpMeth=Interpolation-Use End Values  OutDataType=sfix(16)  OutScaling=2^0  SaturateOnIntegerOverflow=on
  Product : Product  OutDataType=sfix(16)  OutScaling=2^0  SaturateOnIntegerOverflow=on  InputSameDT=on
  Product1 : Product  Orientation=left  OutDataType=sfix(16)  OutScaling=2^0  SaturateOnIntegerOverflow=on  InputSameDT=on
  Tout : Outport  InitialOutput=0
  Nin : Outport  Orientation=left  Port=2  InitialOutput=0
  wires:
  Abs1/1 -> Product1/2
  Abs/1 -> Product1/1
  gear/1 -> Look-Up Table/1
  Tin/1 -> Product/1
  Product/1 -> Tout/1
  Product1/1 -> Nin/1
  Nout/1 -> Abs1/1
  Look-Up Table/1 -> Abs/1, Product/2

== system hil14_mdl_lib/Transmission Model/transmission/Torque Converter ==
  Ne : Inport  OutDataType=sfix(16)  OutScaling=2^0
  Nin : Inport  Port=2  OutDataType=sfix(16)  OutScaling=2^0
  K factor : Lookup  InputValues=speedratio  Table=Kfactor  OutDataType=sfix(16)  OutScaling=2^0  SaturateOnIntegerOverflow=on
  Torque ratio : Lookup  InputValues=speedratio  Table=Torkratio  OutDataType=sfix(16)  OutScaling=2^0  SaturateOnIntegerOverflow=on
  impeller : Fcn  Expr=u^2
  quotient : Product  Inputs=*/  OutDataType=sfix(16)  OutScaling=2^0  SaturateOnIntegerOverflow=on  InputSameDT=on
  speed ratio : Product  Inputs=*/  OutDataType=sfix(16)  OutScaling=2^0  SaturateOnIntegerOverflow=on  InputSameDT=on
  turbine : Product  OutDataType=sfix(16)  OutScaling=2^0  SaturateOnIntegerOverflow=on  InputSameDT=on
  Ti : Outport  InitialOutput=0
  Tt : Outport  Port=2  InitialOutput=0
  wires:
  Nin/1 -> speed ratio/1
  Ne/1 -> quotient/1, speed ratio/2
  turbine/1 -> Tt/1
  impeller/1 -> Ti/1, turbine/1
  speed ratio/1 -> K factor/1, Torque ratio/1
  K factor/1 -> quotient/2
  quotient/1 -> impeller/1
  Torque ratio/1 -> turbine/2

== system hil14_mdl_lib/Transmission Model/transmission/transmission ratio ==
  Tin : Inport  OutDataType=sfix(16)  OutScaling=2^0
  gear : Inport  Port=2  OutDataType=sfix(16)  OutScaling=2^0
  Nout : Inport  Orientation=left  Port=3  OutDataType=sfix(16)  OutScaling=2^0
  Look-Up Table : Lookup  InputValues=[1 2 3 4]  Table=[2.393 1.450 1.000 0.677]  OutDataType=sfix(16)  OutScaling=2^0  SaturateOnIntegerOverflow=on
  Product : Product  OutDataType=sfix(16)  OutScaling=2^0  SaturateOnIntegerOverflow=on  InputSameDT=on
  Product1 : Product  Orientation=left  OutDataType=sfix(16)  OutScaling=2^0  SaturateOnIntegerOverflow=on  InputSameDT=on
  Tout : Outport  InitialOutput=0
  Nin : Outport  Orientation=left  Port=2  InitialOutput=0
  wires:
  gear/1 -> Look-Up Table/1
  Tin/1 -> Product/1
  Product/1 -> Tout/1
  Product1/1 -> Nin/1
  Nout/1 -> Product1/2
  Look-Up Table/1 -> Product/2, Product1/1

== system hil14_mdl_lib/Engine Model/Manifod Model/Intake Manifold Flow/Intake Density ==
  IMP [Bar] : Inport  OutDataType=sfix(16)  OutScaling=2^0
  IMT [C] : Inport  Port=2  OutDataType=sfix(16)  OutScaling=2^0
  Bar to Pascals : Gain  Gain=100000  ParameterDataType=sfix(16)  ParameterScaling=2^0  OutDataType=sfix(16)  OutScaling=2^0
  Constant : Constant  Value=287.05  OutDataType=sfix(16)  OutScaling=2^0
  Constant1 : Constant  Value=273  OutDataType=sfix(16)  OutScaling=2^0
  Display1 : Display
  Product : Product  Inputs=*//  OutDataType=sfix(16)  OutScaling=2^0  RndMeth=Zero
  Sum : Sum  Inputs=|++  OutDataType=sfix(16)  OutScaling=2^0
  Title Block : ni_annotations_lib/Title Block  SystemSampleTime=-1  tx_title=get_param(gcs,'Name')
  Intake Density [Kg/m^3] : Outport  OutDataType=sfix(16)  OutScaling=2^0
  wires:
  Bar to Pascals/1 -> Product/1
  Constant/1 -> Product/3
  IMT [C]/1 -> Sum/1
  Constant1/1 -> Sum/2
  Sum/1 -> Product/2
  IMP [Bar]/1 -> Bar to Pascals/1
  Product/1 -> Display1/1, Intake Density [Kg/m^3]/1

== stateflow chart Transmission Model/shift_logic ==
  settings: updateMethod=DISCRETE  sampleTime=0.04
  state gear_state [parallel]
    settings: executionOrder=1
    state fourth
      entry: gear = 4;
    state second
      entry: gear = 2;
    state third
      entry: gear = 3;
    state first
      entry: gear = 1;
    third -> fourth [order 1] : UP
    second -> third [order 1] : UP
    first -> second : UP
    (default) -> first
    fourth -> third : DOWN
    third -> second [order 2] : DOWN
    second -> first [order 2] : DOWN
  state selection_state [parallel]
    during: CALC_TH;
    settings: executionOrder=2
    state downshifting
    state upshifting
    state steady_state
    (default) -> steady_state
    steady_state -> upshifting [order 1] : [speed > up_th]
    steady_state -> downshifting [order 2] : [speed < down_th]
    upshifting -> steady_state [order 2] : [speed < up_th]
    downshifting -> steady_state [order 2] : [speed > down_th]
    downshifting -> steady_state [order 1] : after(TWAIT,tick)
        | [speed <= down_th]
        | {gear_state.DOWN}
    upshifting -> steady_state [order 1] : after(TWAIT,tick)
        | [speed >= up_th]
        | {gear_state.UP}
  data: speed input double; gear output uint8 [1..4] =1; TWAIT parameter uint8; up_th input double; down_th input double
  data speed settings: units=double
  data gear settings: units=int
  events: DOWN local EITHER_EDGE_EVENT; UP local EITHER_EDGE_EVENT; CALC_TH output FUNCTION_CALL_EVENT
